simulink model "Blood_platelet_Count_V3"  (R2022a)
settings: Solver=VariableStepAuto  StartTime=0.0  StopTime=10.0  RelTol=1e-3
libraries: simulink x9
settings Model: Creator=KVJ RAMAN  LastModifiedBy=KVJ RAMAN

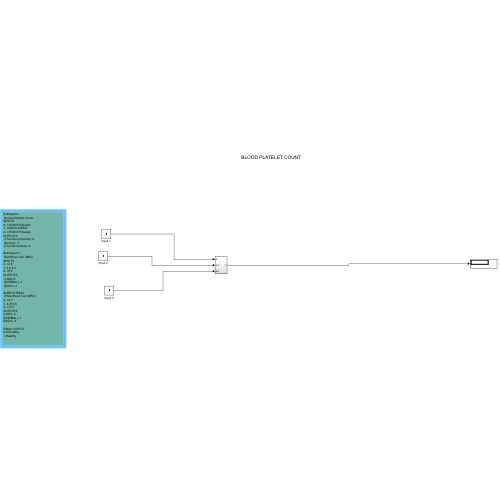
[thumbnail: Simulink's stored preview of the top-level diagram]
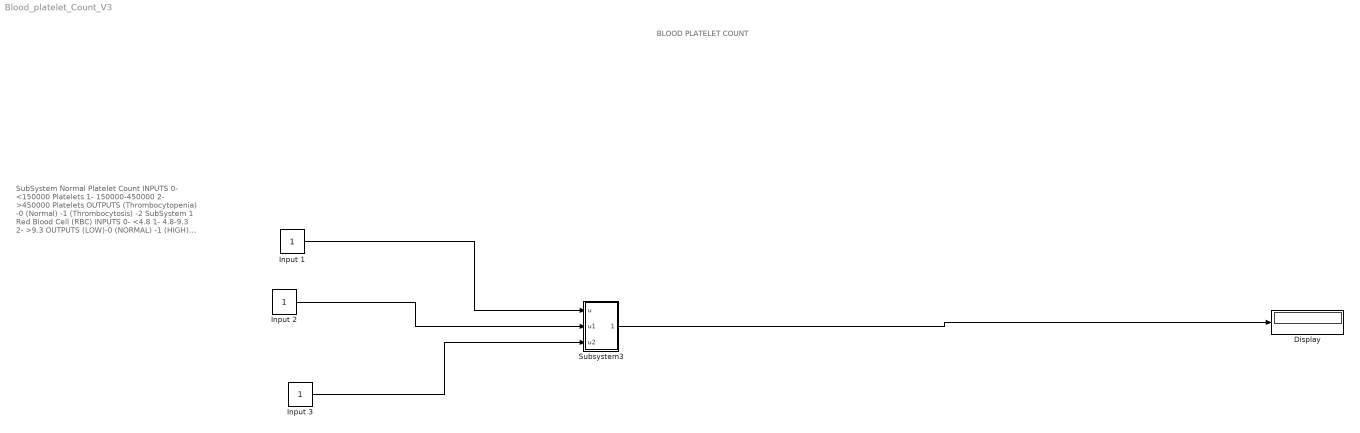
== system Blood_platelet_Count_V3 ==
  note: BLOOD PLATELET COUNT
  note: SubSystem
      |  Normal Platelet Count
      | INPUTS
      | 0- <150000 Platelets
      | 1- 150000-450000
      | 2- >450000 Platelets
      | OUTPUTS
      |  (Thrombocytopenia) -0
      |  (Normal) -1
      |  (Thrombocytosis) -2
      |
      | SubSystem 1
      |  Red Blood Cell (RBC)
      | INPUTS
      | 0- <4.8
      | 1- 4.8-9.3
      | 2- >9.3
      | OUTPUTS
      |  (LOW)-0
      |  (NORMAL) -1
      |  (HIGH) -2
      |
      | SUBSYSTEM 2
      |  White Blood Cell (WBC)
      | 0- <4.0
      | 1- 4.015.5
      | 2- >15.5
      | OUTPUTS
      | (LOW) -0
      | (NORMAL) -1
      | (HIGH) -2
      |
      | FINAL OUTPUT
      | 0-Unhealthy
      | 1-Healthy
  Display : Display
  Input 1 : Constant
  Input 2 : Constant
  Input 3 : Constant
  Subsystem3 : Subsystem
  wires:
  Input 1/1 -> Subsystem3/1(u)
  Input 2/1 -> Subsystem3/2(u1)
  Input 3/1 -> Subsystem3/3(u2)
  Subsystem3/1(Out1) -> Display/1

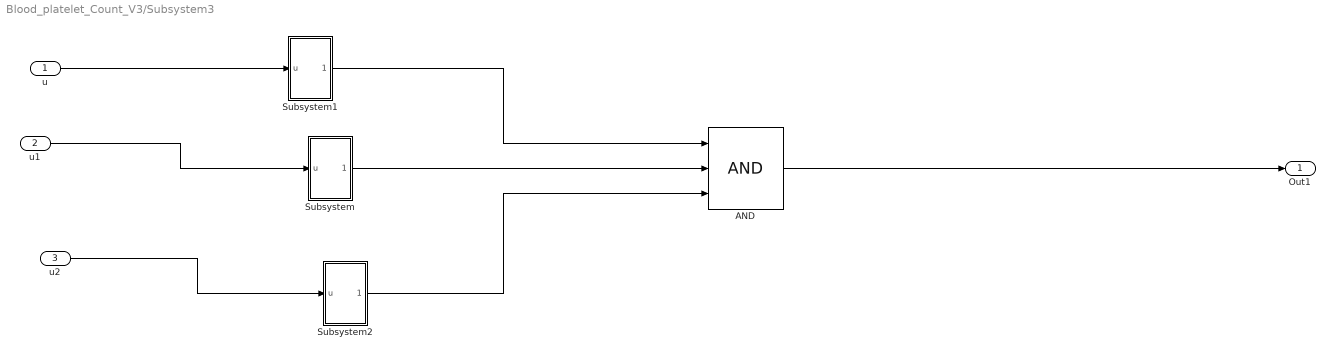
== system Blood_platelet_Count_V3/Subsystem3 ==
  u : Inport
  u1 : Inport  Port=2
  u2 : Inport  Port=3
  AND : Logic  Inputs=3  IconShape=distinctive  AllPortsSameDT=off  OutDataTypeStr=boolean
  Subsystem : Subsystem
  Subsystem1 : Subsystem
  Subsystem2 : Subsystem
  Out1 : Outport
  wires:
  u/1 -> Subsystem1/1(u)
  Subsystem1/1(Out1) -> AND/1
  Subsystem/1(Out1) -> AND/2
  Subsystem2/1(Out1) -> AND/3
  AND/1 -> Out1/1
  u1/1 -> Subsystem/1(u)
  u2/1 -> Subsystem2/1(u)

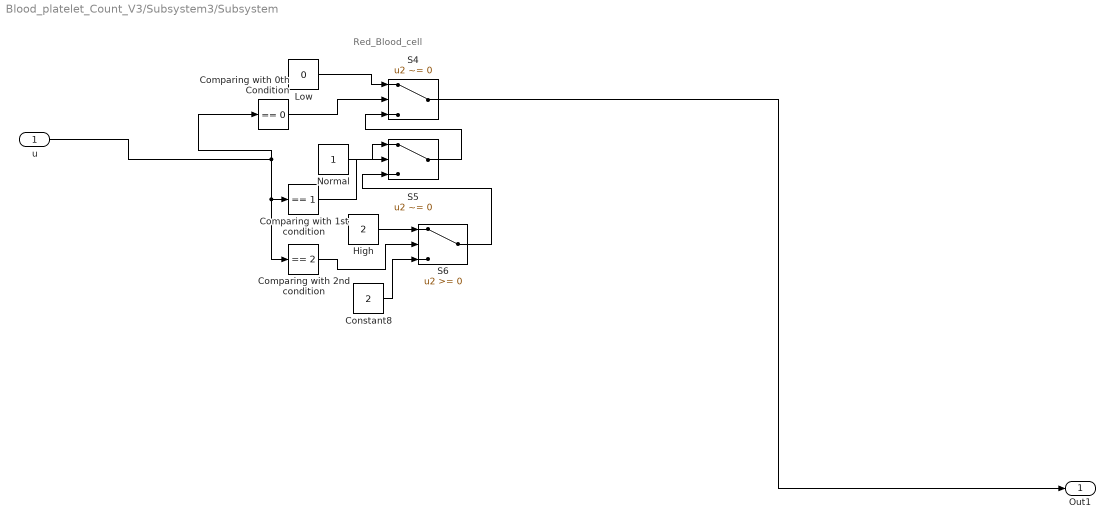
== system Blood_platelet_Count_V3/Subsystem3/Subsystem ==
  note: Red_Blood_cell
  u : Inport
  Comparing with 0th Condition : simulink/Logic and Bit Operations/Compare To Constant  relop===  const=0  OutDataTypeStr=boolean
  Comparing with 1st condition : simulink/Logic and Bit Operations/Compare To Constant  relop===  const=1  OutDataTypeStr=boolean
  "Comparing with 2nd condition " : simulink/Logic and Bit Operations/Compare To Constant  relop===  const=2  OutDataTypeStr=boolean
  Constant8 : Constant  Value=2
  High : Constant  Value=2
  Low : Constant  Value=0
  Normal : Constant
  S4 : Switch  Criteria=u2 ~= 0  SaturateOnIntegerOverflow=off  InputSameDT=off
  S5 : Switch  Criteria=u2 ~= 0  SaturateOnIntegerOverflow=off  InputSameDT=off
  S6 : Switch  SaturateOnIntegerOverflow=off  InputSameDT=off
  Out1 : Outport
  wires:
  Comparing with 1st condition/1 -> S5/2
  "Comparing with 2nd condition "/1 -> S6/2
  S6/1 -> S5/3
  u/1 -> "Comparing with 2nd condition "/1, Comparing with 1st condition/1, Comparing with 0th Condition/1
  Comparing with 0th Condition/1 -> S4/2
  Low/1 -> S4/1
  High/1 -> S6/1
  S5/1 -> S4/3
  Constant8/1 -> S6/3
  Normal/1 -> S5/1
  S4/1 -> Out1/1

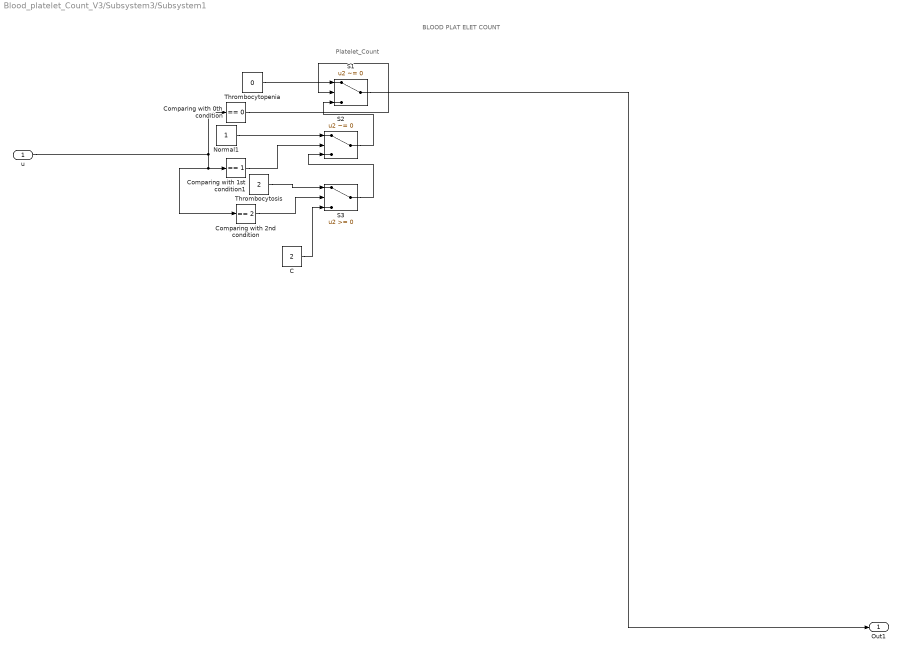
== system Blood_platelet_Count_V3/Subsystem3/Subsystem1 ==
  note: BLOOD PLAT ELET COUNT
  note: Platelet_Count
  u : Inport
  " Comparing with 0th condition" : simulink/Logic and Bit Operations/Compare To Constant  relop===  const=0  OutDataTypeStr=boolean
  C : Constant  Value=2
  Comparing with 1st condition1 : simulink/Logic and Bit Operations/Compare To Constant  relop===  const=1  OutDataTypeStr=boolean
  Comparing with 2nd condition : simulink/Logic and Bit Operations/Compare To Constant  relop===  const=2  OutDataTypeStr=boolean
  Normal1 : Constant
  S1 : Switch  Criteria=u2 ~= 0  SaturateOnIntegerOverflow=off  InputSameDT=off
  S2 : Switch  Criteria=u2 ~= 0  SaturateOnIntegerOverflow=off  InputSameDT=off
  S3 : Switch  SaturateOnIntegerOverflow=off  InputSameDT=off
  Thrombocytopenia : Constant  Value=0
  Thrombocytosis : Constant  Value=2
  Out1 : Outport
  wires:
  S2/1 -> S1/3
  Normal1/1 -> S2/1
  Thrombocytopenia/1 -> S1/1
  Comparing with 2nd condition/1 -> S3/2
  S3/1 -> S2/3
  Comparing with 1st condition1/1 -> S2/2
  C/1 -> S3/3
  u/1 -> " Comparing with 0th condition"/1, Comparing with 2nd condition/1, Comparing with 1st condition1/1
  Thrombocytosis/1 -> S3/1
  " Comparing with 0th condition"/1 -> S1/2
  S1/1 -> Out1/1

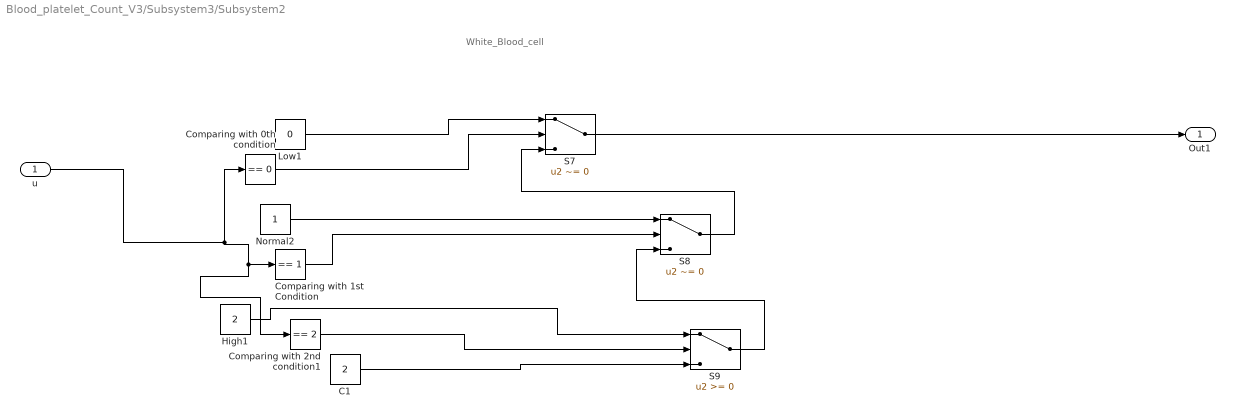
== system Blood_platelet_Count_V3/Subsystem3/Subsystem2 ==
  note: White_Blood_cell
  u : Inport
  C1 : Constant  Value=2
  Comparing with 0th condition : simulink/Logic and Bit Operations/Compare To Constant  relop===  const=0  OutDataTypeStr=boolean
  Comparing with 1st Condition : simulink/Logic and Bit Operations/Compare To Constant  relop===  const=1  OutDataTypeStr=boolean
  Comparing with 2nd condition1 : simulink/Logic and Bit Operations/Compare To Constant  relop===  const=2  OutDataTypeStr=boolean
  High1 : Constant  Value=2
  Low1 : Constant  Value=0
  Normal2 : Constant
  S7 : Switch  Criteria=u2 ~= 0  SaturateOnIntegerOverflow=off  InputSameDT=off
  S8 : Switch  Criteria=u2 ~= 0  SaturateOnIntegerOverflow=off  InputSameDT=off
  S9 : Switch  SaturateOnIntegerOverflow=off  InputSameDT=off
  Out1 : Outport
  wires:
  Comparing with 1st Condition/1 -> S8/2
  Normal2/1 -> S8/1
  u/1 -> Comparing with 2nd condition1/1, Comparing with 1st Condition/1, Comparing with 0th condition/1
  High1/1 -> S9/1
  S7/1 -> Out1/1
  Comparing with 2nd condition1/1 -> S9/2
  Low1/1 -> S7/1
  Comparing with 0th condition/1 -> S7/2
  C1/1 -> S9/3
  S8/1 -> S7/3
  S9/1 -> S8/3
